simulink subsystem "DiffLoss"  (R2022b)
settings: Solver=VariableStepAuto  StartTime=0.0  StopTime=10.0  RelTol=1e-3
undefined symbols (not defined in the file): Diff_EffMap, Diff_Spd_BrkPts, Diff_Trq_BrkPts
libraries: fl_lib x2, nesl_utility x2
settings Model: Creator=Thomas  LastModifiedBy=Thomas

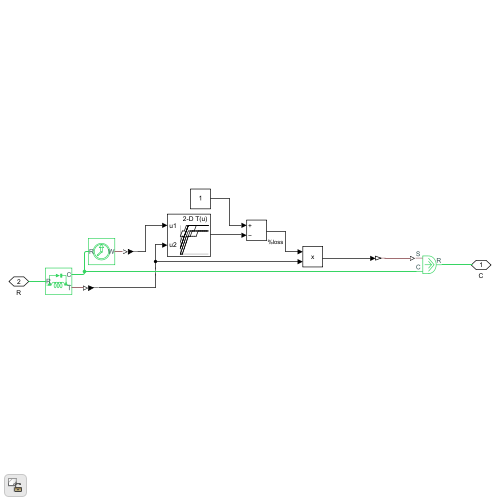
[thumbnail: Simulink's stored preview of the top-level diagram]
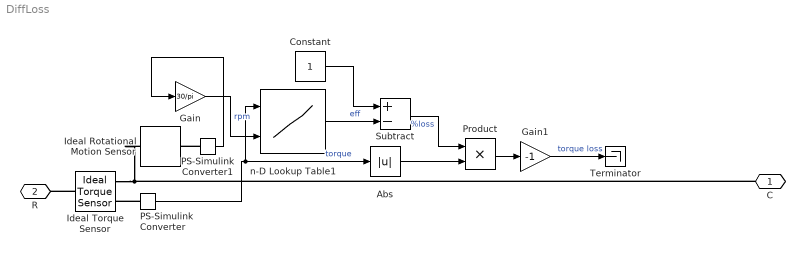
== system DiffLoss ==
  Abs : Abs  SaturateOnIntegerOverflow=off
  Constant : Constant
  Gain : Gain  Gain=30/pi
  Gain1 : Gain  Gain=-1
  Ideal Rotational Motion Sensor : fl_lib/Mechanical/Mechanical Sensors/Ideal Rotational Motion Sensor  reference=foundation.enum.MeasurementReference.absolute  acceleration_port=false  velocity_port=true  position_port=false  wrap_angle=false  offset=0 rad
      settings: InternalSimscapePortConfiguration="{\"Bottom\":[],\"Left\":[{\"id\":\"R\",\"label\":\"R\",\"type\":\"foundation.mechanical.rotational.rotational\"}],\"Right\":[{\"id\":\"W\",\"label\":\"W\",\"type\":\"output\"}],\"Top\":[]}"
  Ideal Torque Sensor : fl_lib/Mechanical/Mechanical Sensors/Ideal Torque Sensor
  PS-Simulink Converter : nesl_utility/PS-Simulink Converter  PhysicalDomain=network_engine_domain  SubClassName=ps_output  LeftPortType=input  RightPortType=output  PseudoPeriodic=off  Frequencies=[]  VectorFormat=inherit  Unit=inherit  AffineConversion=off
  PS-Simulink Converter1 : nesl_utility/PS-Simulink Converter  PhysicalDomain=network_engine_domain  SubClassName=ps_output  LeftPortType=input  RightPortType=output  PseudoPeriodic=off  Frequencies=[]  VectorFormat=inherit  Unit=inherit  AffineConversion=off
  Product : Product
  Subtract : Sum  Inputs=+-
  Terminator : Terminator
  n-D Lookup Table1 : Lookup_n-D  BreakpointsForDimension1=Diff_Trq_BrkPts  BreakpointsForDimension2=Diff_Spd_BrkPts  BreakpointsForDimension3=[5, 7]  Table=Diff_EffMap  ExtrapMethod=Clip  InternalRulePriority=Speed  RndMeth=Simplest
      settings: InputPortMap=u0,u1
  C : PMIOPort  Side=Right
  R : PMIOPort  Port=2  Side=Left
  wires:
  PS-Simulink Converter/1 -> n-D Lookup Table1/1, Abs/1  "torque"
  Constant/1 -> Subtract/1
  Subtract/1 -> Product/1  "%loss"
  n-D Lookup Table1/1 -> Subtract/2  "eff"
  Product/1 -> Gain1/1
  Gain/1 -> n-D Lookup Table1/2  "rpm"
  PS-Simulink Converter1/1 -> Gain/1
  Gain1/1 -> Terminator/1  "torque loss"
  Abs/1 -> Product/2
  connections:
  Ideal Rotational Motion Sensor/LConn1 -- Ideal Torque Sensor/RConn1 -- C/RConn1
  PS-Simulink Converter/LConn1 -- Ideal Torque Sensor/RConn2
  Ideal Torque Sensor/LConn1 -- R/RConn1
  PS-Simulink Converter1/LConn1 -- Ideal Rotational Motion Sensor/RConn1
